simulink model "Baisic_sim"  (R2016a)
settings: Solver=FixedStepAuto  StartTime=0.0  StopTime=10  FixedStep=0.01  RelTol=1e-3
settings Model: Creator=user  LastModifiedBy=user
settings DebuggingCC: InheritedTsInSrcMsg=none  UnknownTsInhSupMsg=none

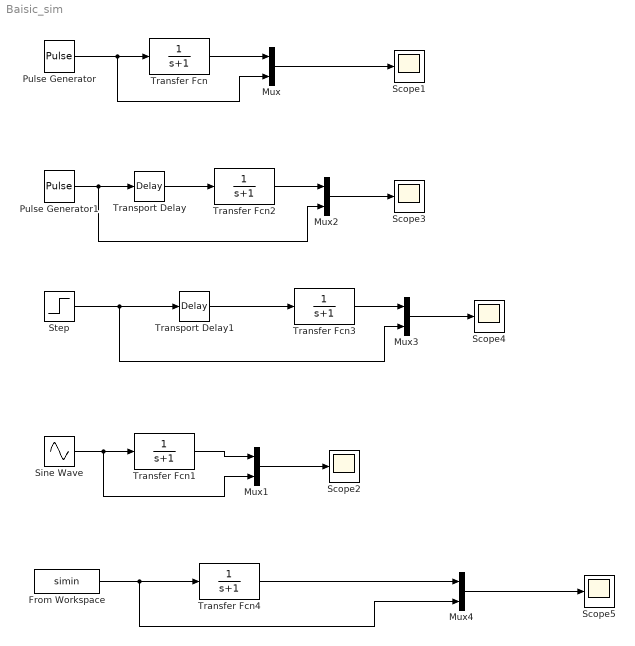
== system Baisic_sim ==
  From Workspace : FromWorkspace  VariableName=simin
  Mux{,1..4} (5 alike) : Mux  Inputs=2
  Pulse Generator : DiscretePulseGenerator  PulseType=Time based  Period=100
  Pulse Generator1 : DiscretePulseGenerator  PulseType=Time based  Period=100
  Scope{1..5} (5 alike) : Scope
  Sine Wave : Sin  Frequency=2*pi
  Step : Step  SampleTime=0
  Transfer Fcn{,1..4} (5 alike) : TransferFcn  Denominator=[1 1]
  Transport Delay : TransportDelay  DelayTime=2
  Transport Delay1 : TransportDelay  DelayTime=2
  wires:
  Pulse Generator/1 -> Mux/2, Transfer Fcn/1
  Transfer Fcn/1 -> Mux/1
  Mux/1 -> Scope1/1
  Sine Wave/1 -> Mux1/2, Transfer Fcn1/1
  Transfer Fcn1/1 -> Mux1/1
  Mux1/1 -> Scope2/1
  Transport Delay/1 -> Transfer Fcn2/1
  Transfer Fcn2/1 -> Mux2/1
  Mux2/1 -> Scope3/1
  Pulse Generator1/1 -> Mux2/2, Transport Delay/1
  Transport Delay1/1 -> Transfer Fcn3/1
  Transfer Fcn3/1 -> Mux3/1
  Mux3/1 -> Scope4/1
  Step/1 -> Mux3/2, Transport Delay1/1
  Transfer Fcn4/1 -> Mux4/1
  Mux4/1 -> Scope5/1
  From Workspace/1 -> Mux4/2, Transfer Fcn4/1
